simulink model "ODE_2"  (R2019b)
settings: Solver=VariableStepAuto  StartTime=0.0  StopTime=40  RelTol=1e-3
settings Model: Creator=ivanl  LastModifiedBy=ivanl

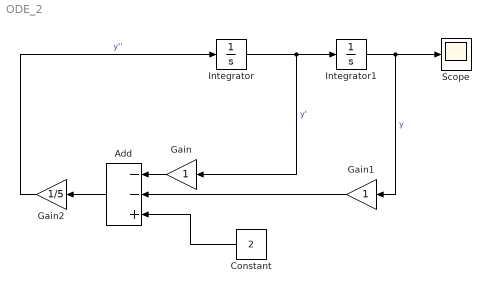
== system ODE_2 ==
  Add : Sum  Inputs=--+
  Constant : Constant  Value=2
  Gain : Gain
  Gain1 : Gain
  Gain2 : Gain  Gain=1/5
  Integrator : Integrator
  Integrator1 : Integrator
  Scope : Scope
  wires:
  Integrator/1 -> Gain/1, Integrator1/1  "y'"
  Gain2/1 -> Integrator/1  "y''"
  Gain/1 -> Add/1
  Gain1/1 -> Add/2
  Integrator1/1 -> Gain1/1, Scope/1  "y"
  Add/1 -> Gain2/1
  Constant/1 -> Add/3
